simulink model "CSRT_LinearTF"  (R2020b)
settings: Solver=FixedStepAuto  StartTime=0.0  StopTime=15  FixedStep=0.01  RelTol=1e-3
values from neighbouring files (symbols this model uses):
  Cas = 8.564    [Exp2_CSRT.m]
libraries: cstblocks x4
settings Model: Creator=franc  LastModifiedBy=franc

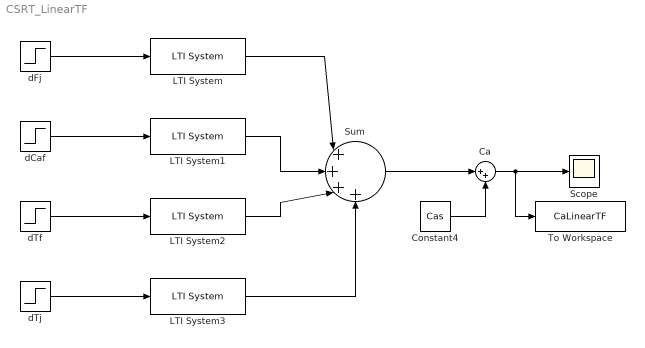
== system CSRT_LinearTF ==
  "                Ca" : Sum  Inputs=|++
  Constant4 : Constant  Value=Cas
  LTI System : cstblocks/LTI System  sys=G  IC=[]
  LTI System1 : cstblocks/LTI System  sys=Gd1  IC=[]
  LTI System2 : cstblocks/LTI System  sys=Gd2  IC=[]
  LTI System3 : cstblocks/LTI System  sys=Gd3  IC=[]
  Scope : Scope
  Sum : Sum  Inputs=|++++
  To Workspace : ToWorkspace  VariableName=CaLinearTF  SaveFormat=Timeseries  SampleTime=-1
  dCaf : Step  Time=0  After=0  SampleTime=0
  dFj : Step  Time=0  After=0.01  SampleTime=0
  dTf : Step  Time=0  After=0  SampleTime=0
  dTj : Step  Time=0  After=0  SampleTime=0
  wires:
  dFj/1 -> LTI System/1
  LTI System/1 -> Sum/1
  dCaf/1 -> LTI System1/1
  dTf/1 -> LTI System2/1
  dTj/1 -> LTI System3/1
  LTI System1/1 -> Sum/2
  LTI System2/1 -> Sum/3
  LTI System3/1 -> Sum/4
  Sum/1 -> "                Ca"/1
  Constant4/1 -> "                Ca"/2
  "                Ca"/1 -> To Workspace/1, Scope/1
